simulink model "VVI_AAI"  (R2022a)
settings: Solver=FixedStepAuto  StartTime=0.0  StopTime=10.0  FixedStep=1e-3  RelTol=1e-3  EnableMultiTasking=on
undefined symbols (not defined in the file): A4, D0, D10, D11, D12, D13, D2, D3, D4, D5, D7, D8, D9, PTA0, PTA1, PTA2, PTB23, PTB9, PTC11, PTC16, PTC3, PTC4, PTD0, PTD1, PTD2, PTD3
libraries: frdmk64flib x15
settings Model: ExtModeTrigDuration=5  Creator=pauls  LastModifiedBy=pauls
settings OptimizationCC: EnhancedBackFolding=on  PassReuseOutputArgsAs=Individual arguments  ZeroExternalMemoryAtStartup=off  ZeroInternalMemoryAtStartup=off  MaxStackSize=64  OptimizeBlockOrder=speed  DifferentSizesBufferReuse=on  OptimizationCustomize=off  EfficientTunableParamExpr=on
settings DebuggingCC: ParameterTunabilityLossMsg=error
settings HardwareCC: ProdBitPerPointer=32  ProdBitPerSizeT=32  ProdBitPerPtrDiffT=32  ProdLargestAtomicInteger=Long  ProdLargestAtomicFloat=Double  ProdWordSize=32  ProdHWDeviceType=ARM Compatible->ARM Cortex
settings SFSimCC: MATLABDynamicMemAlloc=off
settings RTWCC: SystemTargetFile=ert.tlc  HardwareBoard=NXP FRDM-K64F  TLCOptions="-aInlineSetEventsForThisBaseRateFcn=TLC_FALSE -aSuppressMultiTaskScheduler=TLC_FALSE  -aRateBasedStepFcn=0"  TemplateMakefile=ert_default_tmf  Toolchain=GNU Tools for ARM Embedded Processors
settings CodeAppCC: ForceParamTrailComments=on  IgnoreCustomStorageClasses=off  OperatorAnnotations=on  SimulinkDataObjDesc=on  SFDataObjDesc=on  InsertBlockDesc=on
settings ERTTargetCC: ExtModeTransport=4  ExtModeMexFile=sendToCommService

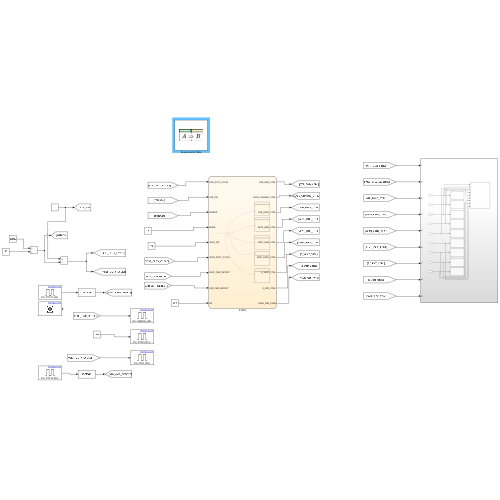
[thumbnail: Simulink's stored preview of the top-level diagram]
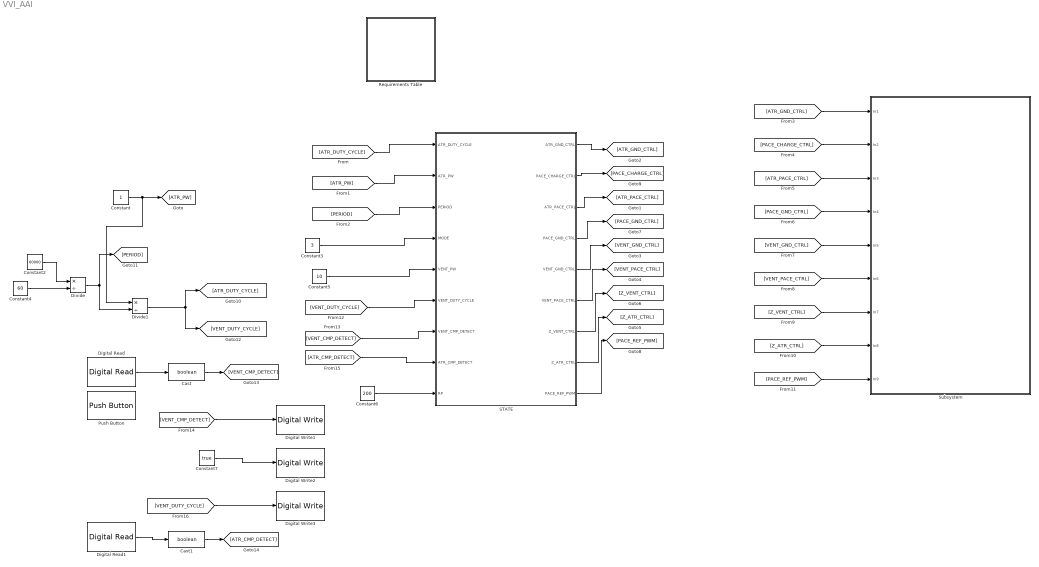
== system VVI_AAI ==
  Cast : DataTypeConversion  OutDataTypeStr=boolean  SaturateOnIntegerOverflow=off  RndMeth=Floor
  Cast1 : DataTypeConversion  OutDataTypeStr=boolean  SaturateOnIntegerOverflow=off  RndMeth=Floor
  Constant : Constant
  Constant2 : Constant  Value=60000
  Constant3 : Constant  Value=3
  Constant4 : Constant  Value=60
  Constant5 : Constant  Value=10
  Constant6 : Constant  Value=200
  Constant7 : Constant  Value=true
  Digital Read : frdmk64flib/Digital Read  Whichpin=PTC11 (A4)  SampleTime=-1
  Digital Read1 : frdmk64flib/Digital Read  Whichpin=PTC16 (D0)  SampleTime=-1
  Digital Write1 : frdmk64flib/Digital Write  Whichpin=GREEN_LED
  Digital Write2 : frdmk64flib/Digital Write  Whichpin=PTD1 (D13)
  Digital Write3 : frdmk64flib/Digital Write  Whichpin=PTA1 (D3)
  Divide : Product  Inputs=*/
  Divide1 : Product  Inputs=*/
  Push Button : frdmk64flib/Push Button  Whichswitch=SW2  SampleTime1=-1
  Requirements Table : Requirements Table  TreatAsAtomicUnit=on
  STATE : Stateflow chart  TreatAsAtomicUnit=on
      settings: PortSchema="{\"entries\":[{\"content\":{\"sides\":[{\"content\":{\"connectorIds\":[\"In2\",\"In3\",\"In4\",\"In5\",\"In6\",\"In7\",\"In1\",\"In9\",\"In8\"]},\"type\":\"ConnectorPlacement.EquallySpacedRectSide\",\"uuid\":\"01118a3a-35ab-415d-a4dc-7a9e5022dc58\"},{\"content\":{\"connectorIds\":[\"Out1\",\"Out2\",\"Out3\",\"Out4\",\"Out5\",\"Out6\",\"Out7\",\"Out8\",\"Out9\"],\"side\":\"RIGHT\"},\"type\":\"ConnectorPlacement.EquallySpacedRectSide\",\"uuid\":\"d119b6db-c579-45b6-8580-2a3960ab3129\"},{\"content\":{\"connectorIds\":[],\"side\":\"TOP\"},\"type\":\"ConnectorPlacement.EquallySpacedRectSide\",\"uuid\":\"18fa5379-1691-4053-811b-8d647a346445\"},{\"content\":{\"connectorIds\":[],\"side\":\"BOTTOM\"},\"type\":\"ConnectorPlacement.EquallySpacedRectSide\",\"uuid\":\"c19ca9f7-b829-4e11-b03e-3e9d42b35795\"}]},\"type\":\"ConnectorPlacement.EquallySpacedConnector\",\"uuid\":\"6e6fa963-33ea-4c14-97b4-73e5587667a9\"}],\"packageUris\":[\"http://schema.mathworks.com/mf0/Connector/R2020b\"],\"version\":\"1.0\"}"
  Subsystem : Subsystem
  wires:
  [ATR_DUTY_CYCLE] -> STATE/2(ATR_DUTY_CYCLE)
  Cast/1 -> [VENT_CMP_DETECT]
  [VENT_GND_CTRL] -> Subsystem/5(In5)
  Constant3/1 -> STATE/5(MODE)
  Constant6/1 -> STATE/8(RP)
  [VENT_PACE_CTRL] -> Subsystem/6(In6)
  [VENT_DUTY_CYCLE] -> STATE/7(VENT_DUTY_CYCLE)
  [PACE_REF_PWM] -> Subsystem/9(In9)
  Constant2/1 -> Divide/1
  [VENT_CMP_DETECT] -> STATE/1(VENT_CMP_DETECT)
  [Z_ATR_CTRL] -> Subsystem/8(In8)
  Constant4/1 -> Divide/2
  [PACE_GND_CTRL] -> Subsystem/4(In4)
  Constant5/1 -> STATE/6(VENT_PW)
  [Z_VENT_CTRL] -> Subsystem/7(In7)
  STATE/4(PACE_GND_CTRL) -> [PACE_GND_CTRL]
  STATE/5(VENT_GND_CTRL) -> [VENT_GND_CTRL]
  [ATR_GND_CTRL] -> Subsystem/1(In1)
  [PACE_CHARGE_CTRL] -> Subsystem/2(In2)
  Divide/1 -> Divide1/2, [PERIOD]
  Divide1/1 -> [VENT_DUTY_CYCLE], [ATR_DUTY_CYCLE]
  [ATR_PACE_CTRL] -> Subsystem/3(In3)
  Constant/1 -> Divide1/1, [ATR_PW]
  STATE/8(Z_ATR_CTRL) -> [Z_ATR_CTRL]
  STATE/6(VENT_PACE_CTRL) -> [VENT_PACE_CTRL]
  STATE/1(ATR_GND_CTRL) -> [ATR_GND_CTRL]
  [ATR_PW] -> STATE/3(ATR_PW)
  STATE/7(Z_VENT_CTRL) -> [Z_VENT_CTRL]
  [VENT_CMP_DETECT] -> Digital Write1/1
  STATE/3(ATR_PACE_CTRL) -> [ATR_PACE_CTRL]
  [PERIOD] -> STATE/4(PERIOD)
  STATE/2(PACE_CHARGE_CTRL) -> [PACE_CHARGE_CTRL]
  Constant7/1 -> Digital Write2/1
  STATE/9(PACE_REF_PWM) -> [PACE_REF_PWM]
  [VENT_DUTY_CYCLE] -> Digital Write3/1
  Cast1/1 -> [ATR_CMP_DETECT]
  Digital Read1/1 -> Cast1/1
  [ATR_CMP_DETECT] -> STATE/9(ATR_CMP_DETECT)
  Digital Read/1 -> Cast/1

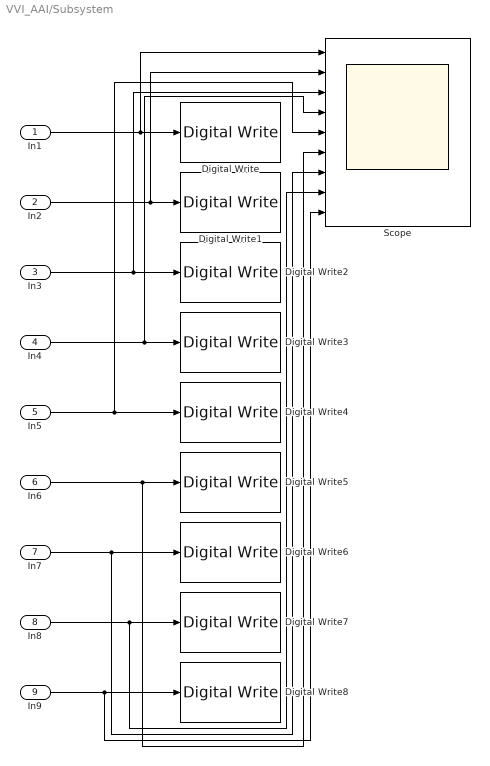
== system VVI_AAI/Subsystem ==
  In1 : Inport
  In2 : Inport  Port=2
  In3 : Inport  Port=3
  In4 : Inport  Port=4
  In5 : Inport  Port=5
  In6 : Inport  Port=6
  In7 : Inport  Port=7
  In8 : Inport  Port=8
  In9 : Inport  Port=9
  Digital Write : frdmk64flib/Digital Write  Whichpin=PTD2 (D11)
  Digital Write1 : frdmk64flib/Digital Write  Whichpin=PTB9 (D2)
  Digital Write2 : frdmk64flib/Digital Write  Whichpin=PTA0 (D8)
  Digital Write3 : frdmk64flib/Digital Write  Whichpin=PTD0 (D10)
  Digital Write4 : frdmk64flib/Digital Write  Whichpin=PTD3 (D12)
  Digital Write5 : frdmk64flib/Digital Write  Whichpin=PTC4 (D9)
  Digital Write6 : frdmk64flib/Digital Write  Whichpin=PTC3 (D7)
  Digital Write7 : frdmk64flib/Digital Write  Whichpin=PTB23 (D4)
  Digital Write8 : frdmk64flib/Digital Write  Whichpin=PTA2 (D5)
  Scope : Scope  NumInputPorts=9
  wires:
  In7/1 -> Scope/7, Digital Write6/1
  In2/1 -> Scope/2, Digital Write1/1
  In6/1 -> Scope/6, Digital Write5/1
  In4/1 -> Scope/4, Digital Write3/1
  In3/1 -> Scope/3, Digital Write2/1
  In9/1 -> Scope/9, Digital Write8/1
  In1/1 -> Scope/1, Digital Write/1
  In8/1 -> Scope/8, Digital Write7/1
  In5/1 -> Scope/5, Digital Write4/1

== stateflow chart VVI_AAI/Requirements Table ==
  (default) -> (junction 1073741860)
  (junction 1073741860) -> (junction 1073741861) : {
      | % SF_REQ_REV_07
      | }
  (junction 1073741861) -> (junction 1073741863) : {
      | % HEADER_ASSIGNMENTS
      |
      | }
  (junction 1073741863) -> (junction 1073741865) : {
      | % START_A_4
      | }
  (junction 1073741865) -> (junction 1073741867) : {
      | }
  (junction 1073741867) -> (junction 1073741869)
  (junction 1073741869) -> (junction 1073741871) : {
      | }
  (junction 1073741871) -> (junction 1073741873) : {
      | % END_A_4
      | }
  (junction 1073741873) -> (junction 1073741898) : {
      | % START_R_1
      | }
  (junction 1073741898) -> (junction 1073741900) : {
      | }
  (junction 1073741900) -> (junction 1073741902) : {
      |
      |
      | }
  (junction 1073741902) -> (junction 1073741904) : {
      | }
  (junction 1073741904) -> (junction 1073741906) : {
      | % END_R_1
      | }

== stateflow chart VVI_AAI/STATE ==
  state AOO [group]
    state CharingC22
      %Capacitor charing state
      ATR_PACE_CTRL = LOW
      VENT_PACE_CTRL = LOW
      PACE_REF_PWM = ATR_DUTY_CYCLE
      PACE_CHARGE_CTRL = HIGH
      %Discharge capacitor
      PACE_GND_CTRL = HIGH
      VENT_PACE_CTRL = LOW
      Z_ATR_CTRL = LOW
      Z_VENT_CTRL = LOW
      ATR_PACE_CTRL = LOW
      ATR_GND_CTRL = LOW
      VENT_GND_CTRL = HIGH
    state AVPacing
      %step 2
      PACE_CHARGE_CTRL = LOW
      PACE_GND_CTRL = HIGH
      ATR_PACE_CTRL = HIGH
      ATR_GND_CTRL = LOW
      Z_ATR_CTRL = LOW
      Z_VENT_CTRL = LOW
      VENT_GND_CTRL = LOW
      VENT_PACE_CTRL = LOW
    AOO.CharingC22 -> AOO.AVPacing : after(PERIOD-ATR_PW, msec)
    AOO.AVPacing -> AOO.CharingC22 : after(ATR_PW, msec)
  state VOO [group]
    state CharingC23
      during:
      %Begin Charging C22 Capacitor
      ATR_PACE_CTRL = LOW
      VENT_PACE_CTRL = LOW
      PACE_REF_PWM = VENT_DUTY_CYCLE
      PACE_CHARGE_CTRL = HIGH
      %Begin Discharging C21 Blocking Capacitor
      PACE_GND_CTRL = HIGH
      VENT_PACE_CTRL = LOW
      Z_ATR_CTRL = LOW
      Z_VENT_CTRL = LOW
      ATR_PACE_CTRL = LOW
      ATR_GND_CTRL = LOW
      VENT_GND_CTRL = HIGH
    state Discharge
      during:
      %Discharge C22 into Ventricle (Vent Pacing)
      %Begin Charging Blocking Capacitor
      PACE_CHARGE_CTRL = LOW
      PACE_GND_CTRL = HIGH
      ATR_PACE_CTRL = LOW
      ATR_GND_CTRL = LOW
      Z_ATR_CTRL = LOW
      Z_VENT_CTRL = LOW
      VENT_GND_CTRL = LOW
      VENT_PACE_CTRL  = HIGH
    VOO.CharingC23 -> VOO.Discharge : after(PERIOD-VENT_PW, msec)
    VOO.Discharge -> VOO.CharingC23 : after(VENT_PW, msec)
  state VVI [group]
    state Inhibit
      %Start preparing for the next pulse
      during:
      %Begin Charging C22 Capacitor
      ATR_PACE_CTRL = LOW
      VENT_PACE_CTRL = LOW
      PACE_REF_PWM = VENT_DUTY_CYCLE
      PACE_CHARGE_CTRL = HIGH
      %Begin Discharging C21 Blocking Capacitor
      PACE_GND_CTRL = HIGH
      VENT_PACE_CTRL = LOW
      Z_ATR_CTRL = LOW
      Z_VENT_CTRL = LOW
      ATR_PACE_CTRL = LOW
      ATR_GND_CTRL = LOW
      VENT_GND_CTRL = HIGH
    state CharingC23
      during:
      %Begin Charging C22 Capacitor
      ATR_PACE_CTRL = LOW
      VENT_PACE_CTRL = LOW
      PACE_REF_PWM = VENT_DUTY_CYCLE
      PACE_CHARGE_CTRL = HIGH
      %Begin Discharging C21 Blocking Capacitor
      PACE_GND_CTRL = HIGH
      VENT_PACE_CTRL = LOW
      Z_ATR_CTRL = LOW
      Z_VENT_CTRL = LOW
      ATR_PACE_CTRL = LOW
      ATR_GND_CTRL = LOW
      VENT_GND_CTRL = HIGH
    state Discharge
      during:
      %Discharge C22 into Ventricle (Vent Pacing)
      %Begin Charging Blocking Capacitor
      PACE_CHARGE_CTRL = LOW
      PACE_GND_CTRL = HIGH
      ATR_PACE_CTRL = LOW
      ATR_GND_CTRL = LOW
      Z_ATR_CTRL = LOW
      Z_VENT_CTRL = LOW
      VENT_GND_CTRL = LOW
      VENT_PACE_CTRL  = HIGH
    VVI.Inhibit -> VVI.CharingC23 : after(RP,msec)
    VVI.Discharge -> VVI.Inhibit : after(VENT_PW, msec)
    (junction 110) -> VVI.Inhibit : [after(PERIOD,msec)]
    VVI.CharingC23 -> (junction 110) [order 2] : [VENT_CMP_DETECT == true]
    VVI.CharingC23 -> VVI.Discharge [order 1] : after(PERIOD-VENT_PW, msec)
  state AAI [group]
    state Inhibit
      during:
      %Capacitor charing state
      ATR_PACE_CTRL = LOW
      VENT_PACE_CTRL = LOW
      PACE_REF_PWM = ATR_DUTY_CYCLE
      PACE_CHARGE_CTRL = HIGH
      %Discharge capacitor
      PACE_GND_CTRL = HIGH
      VENT_PACE_CTRL = LOW
      Z_ATR_CTRL = LOW
      Z_VENT_CTRL = LOW
      ATR_PACE_CTRL = LOW
      ATR_GND_CTRL = LOW
      VENT_GND_CTRL = HIGH
    state AVPacing
      %step 2
      PACE_CHARGE_CTRL = LOW
      PACE_GND_CTRL = HIGH
      ATR_PACE_CTRL = HIGH
      ATR_GND_CTRL = LOW
      Z_ATR_CTRL = LOW
      Z_VENT_CTRL = LOW
      VENT_GND_CTRL = LOW
      VENT_PACE_CTRL = LOW
    state CharingC22
      %Capacitor charing state
      ATR_PACE_CTRL = LOW
      VENT_PACE_CTRL = LOW
      PACE_REF_PWM = ATR_DUTY_CYCLE
      PACE_CHARGE_CTRL = HIGH
      %Discharge capacitor
      PACE_GND_CTRL = HIGH
      VENT_PACE_CTRL = LOW
      Z_ATR_CTRL = LOW
      Z_VENT_CTRL = LOW
      ATR_PACE_CTRL = LOW
      ATR_GND_CTRL = LOW
      VENT_GND_CTRL = HIGH
    AAI.AVPacing -> AAI.Inhibit : after(ATR_PW, msec)
    AAI.Inhibit -> AAI.CharingC22 : after(RP,msec)
    (junction 123) -> AAI.Inhibit : [after(ATR_PW,msec)]
    AAI.CharingC22 -> (junction 123) [order 2] : [ATR_CMP_DETECT == true]
    AAI.CharingC22 -> AAI.AVPacing [order 1] : after(PERIOD-ATR_PW, msec)
  state TEST [group]
    state CharingC23
      %Capacitor charing state
      ATR_PACE_CTRL = LOW
      VENT_PACE_CTRL = LOW
      PACE_REF_PWM = ATR_DUTY_CYCLE
      PACE_CHARGE_CTRL = HIGH
      %Discharge capacitor
      PACE_GND_CTRL = HIGH
      VENT_PACE_CTRL = LOW
      Z_ATR_CTRL = LOW
      Z_VENT_CTRL = LOW
      ATR_PACE_CTRL = LOW
      ATR_GND_CTRL = LOW
      VENT_GND_CTRL = HIGH
    state AVPacing1
      %step 2
      PACE_CHARGE_CTRL = LOW
      PACE_GND_CTRL = HIGH
      ATR_PACE_CTRL = HIGH
      ATR_GND_CTRL = LOW
      Z_ATR_CTRL = LOW
      Z_VENT_CTRL = LOW
      VENT_GND_CTRL = LOW
      VENT_PACE_CTRL = LOW
    TEST.CharingC23 -> AVPacing1 : after(PERIOD-ATR_PW, msec)
    AVPacing1 -> TEST.CharingC23 : after(ATR_PW, msec)
  (junction 37) -> TEST.CharingC23 [order 5]
  (junction 37) -> VVI.CharingC23 [order 3] : [MODE ==3]
  (junction 37) -> AAI.CharingC22 [order 4] : [MODE == 4]
  (junction 37) -> AOO.CharingC22 [order 1] : [MODE ==1]
  (junction 37) -> VOO.CharingC23 [order 2] : [MODE ==2]
  (default) -> (junction 37)
  data: VENT_CMP_DETECT input; HIGH local =true; LOW local =false; ATR_GND_CTRL output; PACE_CHARGE_CTRL output; ATR_PACE_CTRL output; PACE_GND_CTRL output; VENT_GND_CTRL output; VENT_PACE_CTRL output; Z_VENT_CTRL output; Z_ATR_CTRL output; PACE_REF_PWM output; ATR_DUTY_CYCLE input; ATR_PW input; PERIOD input; MODE input; VENT_PW input; VENT_DUTY_CYCLE input; RP input; ATR_CMP_DETECT input
